simulink model "testStateSpace"  (R2017b)
settings: Solver=ode45  StartTime=0.0  StopTime=0.2  MaxStep=0.01  RelTol=1e-3  EnableMultiTasking=on
settings Model: Creator=guillaume.laurent  LastModifiedBy=guillaume.laurent
settings DataIOCC: LimitDataPoints=on  SaveFormat=Array  SignalLoggingSaveFormat=ModelDataLogs
settings OptimizationCC: ExpressionDepthLimit=2147483647  LifeSpan=inf
settings DebuggingCC: UnderspecifiedInitializationDetection=Classic  MergeDetectMultiDrivingBlocksExec=none  SolverPrmCheckMsg=warning  FcnCallInpInsideContextMsg=warning  StateNameClashWarn=warning  StrictBusMsg=Warning  SFUnexpectedBacktrackingDiag=warning  SFNoUnconditionalDefaultTransitionDiag=warning  SFExecutionAtInitializationDiag=none
settings HardwareCC: ProdBitPerPointer=32  ProdBitPerSizeT=32  ProdBitPerPtrDiffT=32  ProdLargestAtomicFloat=None  ProdIntDivRoundTo=Undefined  ProdEndianess=Unspecified  ProdWordSize=32  ProdHWDeviceType=32-bit Generic
settings ModelReferenceCC: PropagateSignalLabelsOutOfModel=off
settings CodeAppCC: StateflowObjectComments=on
settings GRTTargetCC: TargetLangStandard=C89/C90 (ANSI)  GeneratePreprocessorConditionals=Disable all  CombineOutputUpdateFcns=off  GRTInterface=on
settings ConfigComp: CovMetricSettings=dw  CovHtmlReporting=on  CovSaveCumulativeToWorkspaceVar=on  CovSaveSingleToWorkspaceVar=on  CovExternalEMLEnable=off

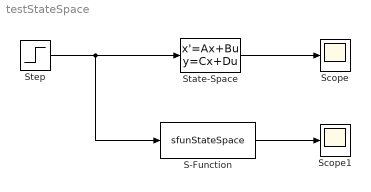
== system testStateSpace ==
  S-Function : S-Function  FunctionName=sfunStateSpace  Parameters="[ -0.09  -0.01 ;  1   ,  0   ]  [  1    -7  ;   0   , -2   ] [  0    2  ;  1   , -5   ] [ -3   0   ;   1   , 0     ]"  SFunctionDeploymentMode=off  EnableBusSupport=off
  Scope : Scope
  Scope1 : Scope
  State-Space : StateSpace  A="[ -0.09  -0.01 ;  1   ,  0   ]"  B="[  1    -7  ;   0   , -2   ]"  C="[  0    2  ;  1   , -5   ]"  D="[ -3   0   ;   1   , 0     ]"  InitialCondition=0
  Step : Step  Time=0.1  Before=[0 0]  After=[1 1]  SampleTime=0
  wires:
  Step/1 -> State-Space/1, S-Function/1
  State-Space/1 -> Scope/1
  S-Function/1 -> Scope1/1
